simulink model "Q2_Part2"  (R2020a)
settings: Solver=VariableStepAuto  StartTime=0.0  StopTime=10.0  RelTol=1e-3
settings Model: Creator=golnazsalehi  LastModifiedBy=golnazsalehi

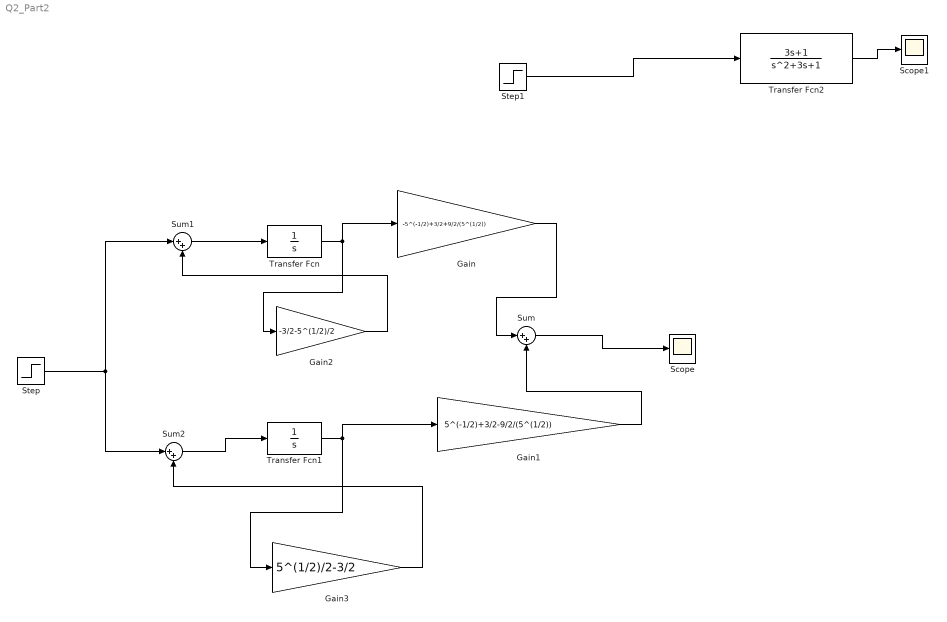
== system Q2_Part2 ==
  Gain : Gain  Gain=-5^(-1/2)+3/2+9/2/(5^(1/2))
  Gain1 : Gain  Gain=5^(-1/2)+3/2-9/2/(5^(1/2))
  Gain2 : Gain  Gain=-3/2-5^(1/2)/2
  Gain3 : Gain  Gain=5^(1/2)/2-3/2
  Scope : Scope
  Scope1 : Scope
  Step : Step  Time=0  SampleTime=0
  Step1 : Step  Time=0  SampleTime=0
  Sum : Sum  Inputs=|++
  Sum1 : Sum  Inputs=|++
  Sum2 : Sum  Inputs=|++
  Transfer Fcn : TransferFcn  Denominator=[1 0]
  Transfer Fcn1 : TransferFcn  Denominator=[1 0]
  Transfer Fcn2 : TransferFcn  Numerator=[3 1]  Denominator=[1 3 1]
  wires:
  Transfer Fcn1/1 -> Gain1/1, Gain3/1
  Gain3/1 -> Sum2/2
  Sum2/1 -> Transfer Fcn1/1
  Gain1/1 -> Sum/2
  Transfer Fcn/1 -> Gain/1, Gain2/1
  Gain2/1 -> Sum1/2
  Sum1/1 -> Transfer Fcn/1
  Gain/1 -> Sum/1
  Step/1 -> Sum2/1, Sum1/1
  Sum/1 -> Scope/1
  Step1/1 -> Transfer Fcn2/1
  Transfer Fcn2/1 -> Scope1/1
